simulink library "RGPadaptCWflight_cl"  (R2018b)
settings: Solver=VariableStepAuto  StartTime=0.0  StopTime=10.0  RelTol=1e-3
undefined symbols (not defined in the file): basisCovNorm, redBasisParaGridLogicIC, sigmaSqColor, size_grid
libraries: filteredPDController_ul x3
settings Model: Creator=mcobb  LastModifiedBy=jdees

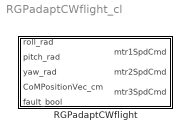
== system RGPadaptCWflight_cl ==
  RGPadaptCWflight : Subsystem

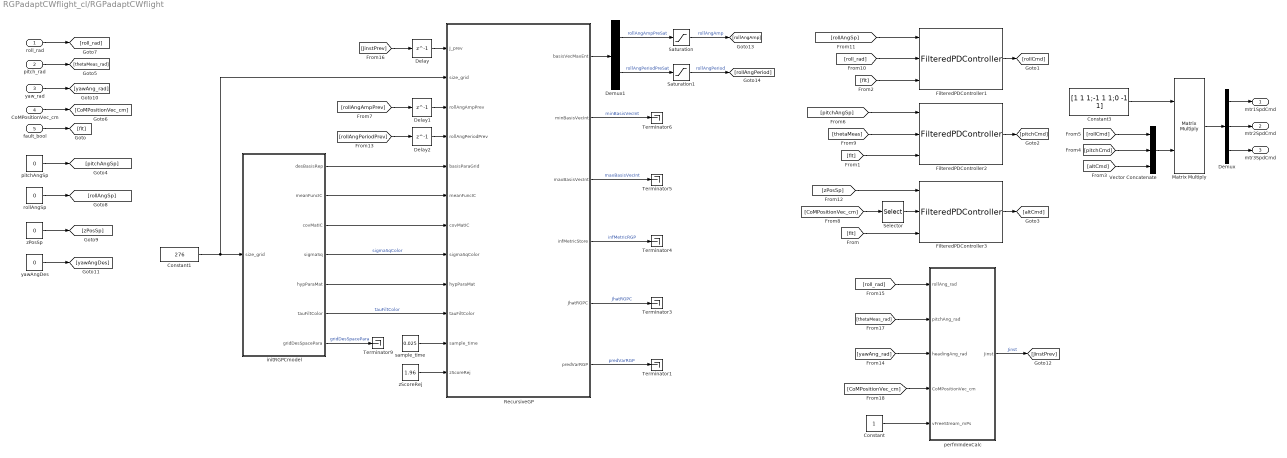
== system RGPadaptCWflight_cl/RGPadaptCWflight ==
  roll_rad : Inport
  pitch_rad : Inport  Port=2
  yaw_rad : Inport  Port=3
  CoMPositionVec_cm : Inport  Port=4
  fault_bool : Inport  Port=5  OutDataTypeStr=boolean
  Constant : Constant
  Constant1 : Constant  Value=276
  Constant3 : Constant  Value=[1 1 1;-1 1 1;0 -1 1]
  Delay : Delay  DelayLength=1
  Delay1 : Delay  DelayLength=1
  Delay2 : Delay  DelayLength=1
  Demux : Demux  Outputs=3
  Demux1 : Demux  Outputs=2
  FilteredPDController1 : filteredPDController_ul/FilteredPDController  enable=on  kp=1  kd=0  timeConstant_s=0.1  intialError=0  initialOutput=0
  FilteredPDController2 : filteredPDController_ul/FilteredPDController  enable=on  kp=1  kd=0  timeConstant_s=0.1  intialError=0  initialOutput=0
  FilteredPDController3 : filteredPDController_ul/FilteredPDController  enable=on  kp=1  kd=0  timeConstant_s=0.1  intialError=0  initialOutput=0
  Matrix Multiply : Product  Multiplication=Matrix(*)
  RecursiveGP : Subsystem
  Saturation : Saturate  UpperLimit=20*pi/180  LowerLimit=1*pi/180
  Saturation1 : Saturate  UpperLimit=10  LowerLimit=4
  Selector : Selector  InputPortWidth=3  IndexOptions=Index vector (dialog)  Indices=3  OutputSizes=1
  Terminator{1,3..6,9} (6 alike) : Terminator
  Vector Concatenate : Concatenate  NumInputs=3
  initRGPCmodel : MATLAB Function  TreatAsAtomicUnit=on
  perfmIndexCalc : MATLAB Function  TreatAsAtomicUnit=on
  pitchAngSp : Constant  Value=0
  rollAngSp : Constant  Value=0
  sample_time : Constant  Value=0.025
  yawAngDes : Constant  Value=0
  zPosSp : Constant  Value=0
  zScoreRej : Constant  Value=1.96
  mtr1SpdCmd : Outport
  mtr2SpdCmd : Outport  Port=2
  mtr3SpdCmd : Outport  Port=3
  wires:
  [rollAngSp] -> FilteredPDController1/1
  FilteredPDController2/1 -> [pitchCmd]
  [altCmd] -> Vector Concatenate/3
  FilteredPDController3/1 -> [altCmd]
  FilteredPDController1/1 -> [rollCmd]
  [flt] -> FilteredPDController3/3
  [flt] -> FilteredPDController1/3
  Selector/1 -> FilteredPDController3/2
  [zPosSp] -> FilteredPDController3/1
  [rollCmd] -> Vector Concatenate/1
  Matrix Multiply/1 -> Demux/1
  Vector Concatenate/1 -> Matrix Multiply/2
  fault_bool/1 -> [flt]
  [pitchCmd] -> Vector Concatenate/2
  [CoMPositionVec_cm] -> Selector/1
  [flt] -> FilteredPDController2/3
  yaw_rad/1 -> [yawAng_rad]
  pitch_rad/1 -> [thetaMeas_rad]
  Constant3/1 -> Matrix Multiply/1
  Demux/2 -> mtr2SpdCmd/1
  Demux/3 -> mtr3SpdCmd/1
  Demux/1 -> mtr1SpdCmd/1
  [pitchAngSp] -> FilteredPDController2/1
  CoMPositionVec_cm/1 -> [CoMPositionVec_cm]
  [thetaMeas] -> FilteredPDController2/2
  roll_rad/1 -> [roll_rad]
  [roll_rad] -> FilteredPDController1/2
  rollAngSp/1 -> [rollAngSp]
  zPosSp/1 -> [zPosSp]
  yawAngDes/1 -> [yawAngDes]
  perfmIndexCalc/1(Jinst) -> [JinstPrev]  "Jinst"
  Delay/1 -> RecursiveGP/1(J_prev)
  [JinstPrev] -> Delay/1
  initRGPCmodel/3(covMatIC) -> RecursiveGP/7(covMatIC)
  initRGPCmodel/4(sigmaSq) -> RecursiveGP/8(sigmaSqColor)  "sigmaSqColor"
  initRGPCmodel/1(desBasisRep) -> RecursiveGP/5(basisParaGrid)
  Demux1/2 -> Saturation1/1  "rollAngPeriodPreSat"
  initRGPCmodel/2(meanFuncIC) -> RecursiveGP/6(meanFuncIC)
  initRGPCmodel/5(hypParaMat) -> RecursiveGP/9(hypParaMat)
  initRGPCmodel/6(tauFiltColor) -> RecursiveGP/10(tauFiltColor)  "tauFiltColor"
  RecursiveGP/1(basisVecMaxEnt) -> Demux1/1
  zScoreRej/1 -> RecursiveGP/12(zScoreRej)
  Constant1/1 -> initRGPCmodel/1(size_grid), RecursiveGP/2(size_grid)
  sample_time/1 -> RecursiveGP/11(sample_time)
  Demux1/1 -> Saturation/1  "rollAngAmpPreSat"
  RecursiveGP/6(predVarRGP) -> Terminator1/1  "predVarRGP"
  RecursiveGP/5(JhatRGPC) -> Terminator3/1  "JhatRGPC"
  RecursiveGP/4(infMetricStore) -> Terminator4/1  "infMetricRGP"
  RecursiveGP/3(maxBasisVecInt) -> Terminator5/1  "maxBasisVecInt"
  RecursiveGP/2(minBasisVecInt) -> Terminator6/1  "minBasisVecInt"
  pitchAngSp/1 -> [pitchAngSp]
  Delay1/1 -> RecursiveGP/3(rollAngAmpPrev)
  Delay2/1 -> RecursiveGP/4(rollAngPeriodPrev)
  [rollAngAmpPrev] -> Delay1/1
  [rollAngPeriodPrev] -> Delay2/1
  initRGPCmodel/7(gridDesSpacePara) -> Terminator9/1  "gridDesSpacePara"
  Saturation/1 -> [rollAngAmp]  "rollAngAmp"
  Saturation1/1 -> [rollAngPeriod]  "rollAngPeriod"
  [roll_rad] -> perfmIndexCalc/1(rollAng_rad)
  [CoMPositionVec_cm] -> perfmIndexCalc/4(CoMPositionVec_cm)
  [yawAng_rad] -> perfmIndexCalc/3(headingAng_rad)
  [thetaMeas_rad] -> perfmIndexCalc/2(pitchAng_rad)
  Constant/1 -> perfmIndexCalc/5(vFreeStream_mPs)

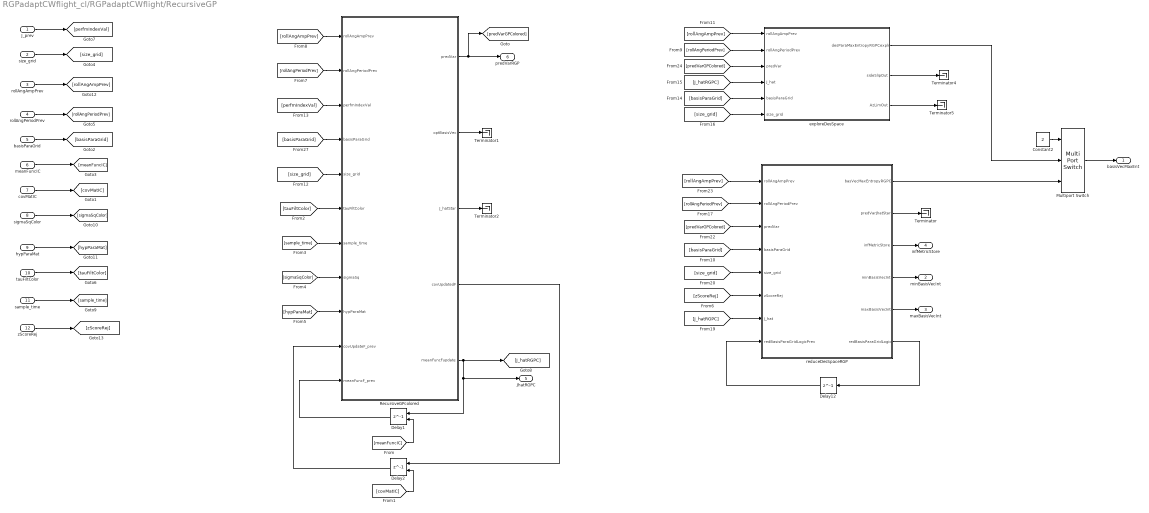
== system RGPadaptCWflight_cl/RGPadaptCWflight/RecursiveGP ==
  J_prev : Inport
  size_grid : Inport  Port=2
  rollAngAmpPrev : Inport  Port=3
  rollAngPeriodPrev : Inport  Port=4
  basisParaGrid : Inport  Port=5
  meanFuncIC : Inport  Port=6
  covMatIC : Inport  Port=7
  sigmaSqColor : Inport  Port=8
  hypParaMat : Inport  Port=9
  tauFiltColor : Inport  Port=10
  sample_time : Inport  Port=11
  zScoreRej : Inport  Port=12
  Constant2 : Constant  Value=2
  Delay1 : Delay  DelayLength=1  InitialConditionSource=Input port  InitialCondition=0.07*ones(size_grid,1)
      settings: InputPortMap=u0,p4
  Delay12 : Delay  DelayLength=1  InitialCondition=redBasisParaGridLogicIC
  Delay2 : Delay  DelayLength=1  InitialConditionSource=Input port  InitialCondition=basisCovNorm*sigmaSqColor
      settings: InputPortMap=u0,p4
  Multiport Switch : MultiPortSwitch  Inputs=2
  RecursiveGPcolored : MATLAB Function  TreatAsAtomicUnit=on
  Terminator{,1..2,4..5} (5 alike) : Terminator
  exploreDesSpace : MATLAB Function  TreatAsAtomicUnit=on
  reduceDesSpaceRGP : MATLAB Function  TreatAsAtomicUnit=on
  basisVecMaxEnt : Outport
  minBasisVecInt : Outport  Port=2  InitialOutput=[1]
  maxBasisVecInt : Outport  Port=3  InitialOutput=size_grid
  infMetricStore : Outport  Port=4  InitialOutput=size_grid
  JhatRGPC : Outport  Port=5  InitialOutput=size_grid
  predVarRGP : Outport  Port=6  InitialOutput=size_grid
  wires:
  basisParaGrid/1 -> [basisParaGrid]
  size_grid/1 -> [size_grid]
  J_prev/1 -> [perfmIndexVal]
  [perfmIndexVal] -> RecursiveGPcolored/3(perfmIndexVal)
  RecursiveGPcolored/4(covUpdatedF) -> Delay2/1
  RecursiveGPcolored/2(optBasisVec) -> Terminator1/1
  RecursiveGPcolored/1(predVar) -> predVarRGP/1, [predVarGPColored]
  [basisParaGrid] -> RecursiveGPcolored/4(basisParaGrid)
  Delay2/1 -> RecursiveGPcolored/10(covUpdateF_prev)
  [size_grid] -> RecursiveGPcolored/5(size_grid)
  Delay1/1 -> RecursiveGPcolored/11(meanFuncF_prev)
  RecursiveGPcolored/3(J_hatStar) -> Terminator2/1
  [predVarGPColored] -> exploreDesSpace/3(predVar)
  [rollAngPeriodPrev] -> exploreDesSpace/2(rollAngPeriodPrev)
  [size_grid] -> exploreDesSpace/6(size_grid)
  [rollAngAmpPrev] -> exploreDesSpace/1(rollAngAmpPrev)
  [basisParaGrid] -> reduceDesSpaceRGP/4(basisParaGrid)
  [size_grid] -> reduceDesSpaceRGP/5(size_grid)
  [predVarGPColored] -> reduceDesSpaceRGP/3(predVar)
  [J_hatRGPC] -> reduceDesSpaceRGP/7(J_hat)
  Constant2/1 -> Multiport Switch/1
  exploreDesSpace/1(desParaMaxEntropyRGPCexplr) -> Multiport Switch/2
  [tauFiltColor] -> RecursiveGPcolored/6(tauFiltColor)
  [sample_time] -> RecursiveGPcolored/7(sample_time)
  [hypParaMat] -> RecursiveGPcolored/9(hypParaMat)
  [sigmaSqColor] -> RecursiveGPcolored/8(sigmaSq)
  reduceDesSpaceRGP/2(predVarJhatStar) -> Terminator/1
  [zScoreRej] -> reduceDesSpaceRGP/6(zScoreRej)
  reduceDesSpaceRGP/3(infMetricStore) -> infMetricStore/1
  [J_hatRGPC] -> exploreDesSpace/4(J_hat)
  reduceDesSpaceRGP/4(minBasisVecInt) -> minBasisVecInt/1
  reduceDesSpaceRGP/5(maxBasisVecInt) -> maxBasisVecInt/1
  Delay12/1 -> reduceDesSpaceRGP/8(redBasisParaGridLogicPrev)
  exploreDesSpace/2(sideSlipOut) -> Terminator4/1
  exploreDesSpace/3(AzLimOut) -> Terminator5/1
  [basisParaGrid] -> exploreDesSpace/5(basisParaGrid)
  rollAngAmpPrev/1 -> [rollAngAmpPrev]
  rollAngPeriodPrev/1 -> [rollAngPeriodPrev]
  [rollAngPeriodPrev] -> RecursiveGPcolored/2(rollAngPeriodPrev)
  [rollAngPeriodPrev] -> reduceDesSpaceRGP/2(rollAngPeriodPrev)
  reduceDesSpaceRGP/6(redBasisParaGridLogic) -> Delay12/1
  [rollAngAmpPrev] -> RecursiveGPcolored/1(rollAngAmpPrev)
  reduceDesSpaceRGP/1(basVecMaxEntropyRGPC) -> Multiport Switch/3
  Multiport Switch/1 -> basisVecMaxEnt/1
  RecursiveGPcolored/5(meanFuncFupdate) -> JhatRGPC/1, Delay1/1, [J_hatRGPC]
  [meanFuncIC] -> Delay1/2
  [covMatIC] -> Delay2/2
  meanFuncIC/1 -> [meanFuncIC]
  covMatIC/1 -> [covMatIC]
  tauFiltColor/1 -> [tauFiltColor]
  sample_time/1 -> [sample_time]
  sigmaSqColor/1 -> [sigmaSqColor]
  hypParaMat/1 -> [hypParaMat]
  zScoreRej/1 -> [zScoreRej]
  [rollAngAmpPrev] -> reduceDesSpaceRGP/1(rollAngAmpPrev)

== matlab function RGPadaptCWflight_cl/RGPadaptCWflight/perfmIndexCalc ==
  data: Jinst output; rollAng_rad input; pitchAng_rad input; headingAng_rad input; CoMPositionVec_cm input; vFreeStream_mPs input
function Jinst   = objFuncCalc(rollAng_rad,... 
    pitchAng_rad,headingAng_rad,CoMPositionVec_cm,vFreeStream_mPs)

% Calculation of zenith angle
zenithAng_rad = pi/2 - atan2((CoMPositionVec_cm(1)^2-CoMPositionVec_cm(2)^2)^0.5,CoMPositionVec_cm(3));

% These are model parameters for 1/100-scale BAT model
radModel = 0.025;           % Radius of scaled model of BAT
Aref = pi*radModel^2;       % Reference area for the BAT
volDispBAT = 0.000282185242;      % Volume displaced by scaled model of BAT
massModel   = 253/1000;            % Mass of scaled model of BAT (kg)
Cp = 0.45;      % Power coefficient of the turbine (theoretical limit = 0.59)
rhoWat = 1000;     % Density of water
Cla = 12.3;     % Lift sensitivity
Cl0 = 0.75;     % Lift - constant offset
Cda = -10.1;    % Draf sensitivity
Cd0 = 0.809;    % Drag - constant offset

% Calculation of apparent wind velocity
vApp_mPs = 1;

liftForce = 0.5*rhoWat*vApp_mPs^2*Aref*((Cl0+Cla*pitchAng_rad));
dragForce = (Cd0+Cda*pitchAng_rad);
buoyForce = 1000*9.8*volDispBAT-massModel*9.8;

tetherTen = liftForce*cos(zenithAng_rad-pitchAng_rad) + dragForce*sin(zenithAng_rad-pitchAng_rad) + buoyForce*cos(zenithAng_rad);

instPower = 0.5*rhoWat*vApp_mPs^3*Aref*Cp;
instPowerFreeStream = 0.5*rhoWat*vFreeStream_mPs^3*Aref*Cp;

% Objective function structure for stationary flight
Jinst = (instPower-tetherTen)/instPowerFreeStream;

== matlab function RGPadaptCWflight_cl/RGPadaptCWflight/RecursiveGP/RecursiveGPcolored ==
  settings: updateMethod=DISCRETE  sampleTime=sample_time
  data: rollAngAmpPrev input; rollAngPeriodPrev input; perfmIndexVal input; basisParaGrid input; size_grid input; predVar output size=[size_grid 1]; optBasisVec output; J_hatStar output; covUpdatedF output size=[size_grid size_grid]; meanFuncFupdate output; tauFiltColor input; sample_time input; sigmaSq input; hypParaMat input; covUpdateF_prev input size=[size_grid size_grid]; meanFuncF_prev input
function [predVar,optBasisVec,J_hatStar,covUpdatedF,... 
    meanFuncFupdate]  = RecursiveGPcolored(rollAngAmpPrev,rollAngPeriodPrev,perfmIndexVal,basisParaGrid,size_grid,... 
    tauFiltColor,sample_time,sigmaSq,hypParaMat,...
    covUpdateF_prev,meanFuncF_prev)
% Preallocation, which may not actually be required here. 
predVar = ones(size_grid,1);
stateTransMat = ones(size_grid,size_grid);

% Convert continuous time time constant for colored noise to a discrete
% time number. This equation was derived by solving a discrete time
% approximation of a continuous-time filter.
discTimeFiltCnst = sample_time/(tauFiltColor+sample_time);

%-------------------------------------------------------------------------
    desParaCur = [rollAngAmpPrev rollAngPeriodPrev];
    responseCurr = perfmIndexVal;
    
    covCurPara = zeros(1,size_grid);
    for ii = 1:size_grid
        covCurPara(1,ii) = covFuncEval(desParaCur,basisParaGrid(ii,:),hypParaMat,sigmaSq);
    end 
    covCurrPoint = covFuncEval(desParaCur,desParaCur,hypParaMat,sigmaSq);
    
    distCur2Grid = zeros(size_grid,1);
    for ii = 1:size_grid
        distCur2Grid(ii,1) = sqrt((desParaCur(1,1)-basisParaGrid(ii,1))^2 + (desParaCur(1,2)-basisParaGrid(ii,2))^2);
    end 
    [~,firstDistIndex] = min(distCur2Grid);

    % The observation matrix is all zeros and a one at the location of the
    % current parameter. This is J_t in the RGP paper
    covUpdateVecColored = zeros(1,size_grid);
    covUpdateVecColored(firstDistIndex) = 1;

    % Mean approximation at the current point
        meanFuncPredCurPt = covUpdateVecColored*meanFuncF_prev;
        obsMat = covUpdateVecColored;

        I_mat = eye(size_grid);   
    % The states for this Kalman filter are the mean function approximation
    % at the basis vector locations. In a application, where there is no
    % temporal variation in the instantaneous objective function, the state
    % transition matrix is simply the identity matrix. 
        stateTransMat = eye(size_grid);
        
        colNoisObsMat = covUpdateVecColored;
           
        colNoisTransMat = (1-discTimeFiltCnst);
        
        % Adjusted observation matrix to consider colored noise
        Hprime = obsMat*stateTransMat - colNoisTransMat*colNoisObsMat;
        
        % Covariance of the current point
        covUpdatedP = covUpdateVecColored*covUpdateF_prev*covUpdateVecColored';
        
        % Kalman gain for measurement differencing approach for Kalman
        % filter. 
        kalGainMatrixNew = covUpdateF_prev*Hprime'*((covUpdatedP + sigmaSq)^(-1));
        
        % Mean and covariance function update. This is just the update step
        % of the Kalman filter
        meanFuncFupdate = meanFuncF_prev + kalGainMatrixNew*(responseCurr - meanFuncPredCurPt);
        covUpdatedF = (I_mat - kalGainMatrixNew*Hprime)*covUpdateF_prev*(I_mat - kalGainMatrixNew*Hprime)';

        % Prediction variance calculation
        predVar = diag(covUpdatedF);
        [J_hatStar,minPerfmVal_index] = min(meanFuncFupdate);
        optBasisVec = basisParaGrid(minPerfmVal_index,:);       
end 

%--------------------------------------------------------------------------    
function [covFuncValue] = covFuncEval(designPt1,designPt2,hypParaMat,noiseVar)
%     covFuncValue = noiseVar*exp(-1/(2*theta^2)*(abs(designPt1-designPt2))^2);
    covFuncValue = noiseVar*exp(-0.5*(designPt1-designPt2)*inv(hypParaMat)*(designPt1-designPt2)');
end

== matlab function RGPadaptCWflight_cl/RGPadaptCWflight/RecursiveGP/exploreDesSpace ==
  settings: updateMethod=DISCRETE  sampleTime=sample_time
  data: desParaMaxEntropyRGPCexplr output; rollAngAmpPrev input; rollAngPeriodPrev input; sideSlipOut output; predVar input size=[size_grid 1]; J_hat input; basisParaGrid input; size_grid input; AzLimOut output
function [desParaMaxEntropyRGPCexplr,sideSlipOut,AzLimOut] = Reduce(rollAngAmpPrev,rollAngPeriodPrev,predVar,J_hat,basisParaGrid,size_grid)

    % This block simply selects the basis vector that maximizes prediction
    % variance. Essentially, this just doesn't include design space
    % reduction.

    dist_update = zeros(size_grid,1);
    [J_hatStar,idx_JhatStar] = min(J_hat);
    
    prevDesPara = [rollAngAmpPrev rollAngPeriodPrev];
    
for c4 = 1:size_grid
    dist_update(c4,1) = sqrt((prevDesPara(1,1)-basisParaGrid(c4,1))^2 + (prevDesPara(1,2)-basisParaGrid(c4,2))^2);
end

    [valMaxEntropy,maxEntropyIndex] = max(predVar.*exp(-100*dist_update.^2));
%     [valMaxEntropy,thetaMaxEntropyIndex] = max(predVar(min_theta_int:max_theta_int));
    desParaMaxEntropyRGPCexplr = basisParaGrid(maxEntropyIndex,:);
    sideSlipOut = desParaMaxEntropyRGPCexplr(1,1);
    AzLimOut = desParaMaxEntropyRGPCexplr(1,2);

== matlab function RGPadaptCWflight_cl/RGPadaptCWflight/RecursiveGP/reduceDesSpaceRGP ==
  settings: updateMethod=DISCRETE  sampleTime=sample_time
  data: rollAngAmpPrev input; rollAngPeriodPrev input; basVecMaxEntropyRGPC output; predVarJhatStar output; infMetricStore output size=[size_grid 1]; minBasisVecInt output; maxBasisVecInt output; predVar input size=[size_grid 1]; basisParaGrid input size=[size_grid 2]; size_grid input; zScoreRej input; J_hat input; redBasisParaGridLogicPrev input; redBasisParaGridLogic output size=[size_grid 2]
function [basVecMaxEntropyRGPC,predVarJhatStar,infMetricStore,minBasisVecInt,... 
    maxBasisVecInt,redBasisParaGridLogic] = ReduceColored(rollAngAmpPrev,rollAngPeriodPrev,predVar,basisParaGrid,... 
    size_grid,zScoreRej,J_hat,redBasisParaGridLogicPrev)
    
    prevDesParam = [rollAngAmpPrev rollAngPeriodPrev];
    
    checkLoop = 0;
%     basisVecMinCheck = [10*ones(size_grid,1) 10*ones(size_grid,1)]';
%     basisVecMaxCheck = [-10*ones(size_grid,1) -10*ones(size_grid,1)]';
    
%     zScoreDesSpace = ones(size_grid,1);
    redBasisParaGridLogic = redBasisParaGridLogicPrev;
    [J_hatStar,maxJhatIndex] = max(J_hat);
    predVarJhatStar = predVar(maxJhatIndex);
    
    [basisIndRedSpace,~] = find(redBasisParaGridLogicPrev(:,1));
    reducedDesSpacePrev = basisParaGrid(basisIndRedSpace,:);
    
% % Design space reduction here is done based on hypothesis testing    
%     for jj = 1:size_grid 
%         zScoreDesSpace(jj) = (J_hat(jj)-J_hatStar)/sqrt(predVar(jj) + predVarJhatStar);
%     end 
%     
%     for ii = 1:size_grid
%         if zScoreDesSpace(ii) <= zScoreRej && zScoreDesSpace(ii) >= -zScoreRej
%             [logic,index] = ismember(basisParaGrid(ii,:),reducedDesSpacePrev,'rows');
%             if logic == 1
%                 redBasisParaGridLogic(ii,:) = [1 1];
%                 check = check + 1;
%             else 
%                 redBasisParaGridLogic(ii,:) = [0 0];
%             end
%         else
%             redBasisParaGridLogic(ii,:) = [0 0];
%         end
%     end
        
    
%         
% Rejection here is done based error bars placed on mean function
% approximation at basis vector locations. The error bars are generated by:
% J_hat +/- 1.96*sigma which corresponds to 95%)

    meanFuncUpperErrorBar = J_hat + zScoreRej*sqrt(predVar);
    meanFuncLowerErrorBar = J_hat - zScoreRej*sqrt(predVar);
    
    meanFuncStarLowerErrorBar = meanFuncLowerErrorBar(maxJhatIndex);
    for ii = 1:size_grid
        if meanFuncUpperErrorBar(ii) >= meanFuncStarLowerErrorBar
            [logic,index] = ismember(basisParaGrid(ii,:),reducedDesSpacePrev,'rows');
            if logic == 1
                redBasisParaGridLogic(ii,:) = [1 1];
            else 
                redBasisParaGridLogic(ii,:) = [0 0];
            end
        else 
            redBasisParaGridLogic(ii,:) = [0 0];
        end
    end
    
%     [~, minBasisVecInt] = min(basisVecMinCheck);
%     [~, maxBasisVecInt] = max(basisVecMaxCheck);
    % This is a patch to avoid taking the max or min of something with zero
    % length
    if sum(redBasisParaGridLogic(:,1)) <= 10
        redBasisParaGridLogic = redBasisParaGridLogicPrev;
    end 

    [basisIndRedSpace,~] = find(redBasisParaGridLogic(:,1));
    minBasisVecInt = min(basisIndRedSpace);
    maxBasisVecInt = max(basisIndRedSpace);

    
    reducedDesSpace = redBasisParaGridLogic.*basisParaGrid;
    
    dist_update = zeros(size_grid,1);
    for c4 = 1:size_grid
        if redBasisParaGridLogic(c4,1) == 1 && redBasisParaGridLogic(c4,2) == 1
            dist_update(c4,1) = sqrt((prevDesParam(1,1)-basisParaGrid(c4,1))^2 + (prevDesParam(1,2)-basisParaGrid(c4,2))^2);
        else 
            dist_update(c4,1) = 0;
        end
    end 
        
    if sum(redBasisParaGridLogic(:,1)) <= 10
        if minBasisVecInt < size_grid
            basVecMaxEntropyRGPC = basisParaGrid(minBasisVecInt+1,:);
        else 
            basVecMaxEntropyRGPC = basisParaGrid(minBasisVecInt,:);
        end 
        infMetricStore = zeros(size_grid,1);
    else 
%         [valMaxEntropy,thetaMaxEntropyIndex] = max(predVar(min_theta_int:max_theta_int).*exp(-100*dist_update.^2));
%         [valMaxEntropy,thetaMaxEntropyIndex] = max(predVar(min_theta_int:max_theta_int));
        predVarReducedDesSpace = predVar.*redBasisParaGridLogic(:,1);
        [valMaxEntropy,basVecMaxEntropyIndex] = max(predVarReducedDesSpace.*exp(-75*dist_update.^2));

%           % Probability of improvement acquisition function 
%           gammaDesSpace = (J_hatStar - J_hat)./predVar;
%           mu = 0;       % Standard normal distribution mean
%           sigma = 1;    % Standard normal distribution standard deviation
%           probImproveDesign = cdf('Normal',gammaDesSpace,mu,sigma);
%           [valProbImprove,thetaMaxEntropyIndex] = max(probImproveDesign(min_theta_int:max_theta_int));

%         % Lower confidence bound acquisition function
%         lowConfBound = J_hat - 2*predVar; % 2 corresponds to 95% confidence (I think)
%         [valLowConfBound,thetaMaxEntropyIndex] = min(lowConfBound);
%         
        basVecMaxEntropyRGPC = basisParaGrid(basVecMaxEntropyIndex,:);
        infMetricStore = predVar;
    end 

    
% dist_update = zeros(size_grid,1);
% 
% for c4 = 1:size_grid
%     dist_update(c4,1) = abs(theta_prev-theta_grid(c4));
% end
% 
%     [valMaxEntropy,thetaMaxEntropyIndex] = max(predVar.*exp(-100*dist_update.^2));
% %     [valMaxEntropy,thetaMaxEntropyIndex] = max(predVar(min_theta_int:max_theta_int));
%     thetaMaxEntropy = theta_grid(thetaMaxEntropyIndex);
%     
% 
% %----------------------------------------------------------------------------
% theta_min_vec = 10*ones(size_grid,1);
% theta_max_vec = -10*ones(size_grid,1);
% 
% minJhat= min(J_hat);
% 
% if minJhat <= 0.001
%     min_theta_int = 1;
%     max_theta_int = size_grid;
%     min_theta = min(theta_grid);
%     max_theta = max(theta_grid);
%     
%     zScoreDesSpace = ones(276,1);
% else 
%     zScoreDesSpace = (J_hat-J_hatStar)./predVar;
%     
%     for i = 1:size_grid
%         if abs(zScoreDesSpace(i)) <= 1.96
%             if theta_grid(i) >= theta_min_prev && theta_grid(i) <= theta_max_prev
%                 theta_min_vec(i,1) =  theta_grid(i);
%                 
%                 theta_max_vec(i,1) = theta_grid(i);
%                 
%                 check = check + 1;
%             end
%         end
%     end
%     
%     [min_theta, min_theta_int] = min(theta_min_vec(:,1));
%     [max_theta, max_theta_int] = max(theta_max_vec(:,1));
%     
%     if max_theta == -10     %   Couldn't find a grid point other than theta_hat_star that could possibly be optimal
%         max_theta = theta_max_prev;         %   Was theta_max_prev
%     end
%     
%     if min_theta == 10      %   Couldn't find a grid point other than theta_hat_star that could possibly be optimal
%         min_theta = theta_min_prev;         %   Was theta_min_prev
%     end
% end 
% 
% theta_max_original = max(theta_grid);
% theta_min_original = min(theta_grid);
% design_space_fullsize = abs(theta_max_original - theta_min_original);
% 
% design_space_size = abs(max_theta - min_theta);
% 
% design_space_percentage = design_space_size/design_space_fullsize;
% 
% 
% dist_update = zeros(max_theta_int-min_theta_int+1,1);
% 
% for c4 = 1:max_theta_int-min_theta_int+1
%     if max_theta_int == size_grid && min_theta_int == 1
%         index = c4;
%     else
%         index = min_theta_int + c4 -1;
%     end
%     
%     dist_update(c4,1) = abs(theta_prev-theta_grid(index));
% end
% 
% if design_space_percentage < 0.01
%     thetaMaxEntropy = min_theta;
% else 
%     [valMaxEntropy,thetaMaxEntropyIndex] = max(predVar(min_theta_int:max_theta_int).*exp(-100*dist_update.^2));
% %     [valMaxEntropy,thetaMaxEntropyIndex] = max(predVar(min_theta_int:max_theta_int));
%     thetaMaxEntropy = theta_grid(thetaMaxEntropyIndex + min_theta_int -1);
% end 
%

== matlab function RGPadaptCWflight_cl/RGPadaptCWflight/initRGPCmodel ==
  data: desBasisRep output; meanFuncIC output; covMatIC output; size_grid input; sigmaSq output; hypParaMat output; tauFiltColor output; gridDesSpacePara output
function [desBasisRep,meanFuncIC,covMatIC,sigmaSq,hypParaMat,... 
    tauFiltColor,gridDesSpacePara]  = RGPinit(size_grid)

desBasisRep = zeros(size_grid,2);
covMatIC = zeros(size_grid,size_grid);

% Initialize the mean function approximation
meanFuncIC = 0.07*ones(size_grid,1);

% Basis vectors for roll period (in seconds)
lenRollPeriodPts = 20;
rollPeriodMin = 4;    
rollPeriodMax = 10;
rollPeriodDesPts = linspace(rollPeriodMin,rollPeriodMax,lenRollPeriodPts);

% Basis vectors for roll angle amplitude
lenRollAmp = 41;
rollAmpMin = 0*(pi/180);
rollAmpMax = 20*(pi/180);
rollAmpDesPts = linspace(rollAmpMin,rollAmpMax,lenRollAmp);

% This vector is used to keep up with what the basis vectors were in the
% .mat file that is generated for the collected data.
gridDesSpacePara = [lenRollAmp rollAmpMin rollAmpMax lenRollPeriodPts rollPeriodMin rollPeriodMax];

count = 1;
for ii = 1:lenRollPeriodPts
    for jj = 1:lenRollAmp
        desBasisRep(count,:) = [rollPeriodDesPts(ii) rollAmpDesPts(jj)];
        count = count +1;
    end 
end 

hypParaMat = [0.02^2 0; 0 0.02^2];
sigmaSq = 0.020;
tauFiltColor = 0.25;

for ii = 1:size_grid
    for jj = 1:size_grid
%         basisCov(ii,jj) = covFuncEval(theta_grid(ii),theta_grid(jj),hypPara); 
        covMatIC(ii,jj) = sigmaSq*exp(-0.5*(desBasisRep(ii,:)-desBasisRep(jj,:))*inv(hypParaMat)*(desBasisRep(ii,:)-desBasisRep(jj,:))');
    end 
end
